simulink model "system_identification"  (R2024b)
settings: Solver=VariableStepAuto  StartTime=0.0  StopTime=1000  RelTol=1e-3
model workspace (MAT data in the model file):
  d = 0.5
  eps = 1
values from neighbouring files (symbols this model uses):
  s_L = slipRange(j)    [identify_system.m]
  s_R = slipRange(i)    [identify_system.m]
settings Model: Creator=radnor  LastModifiedBy=radnor

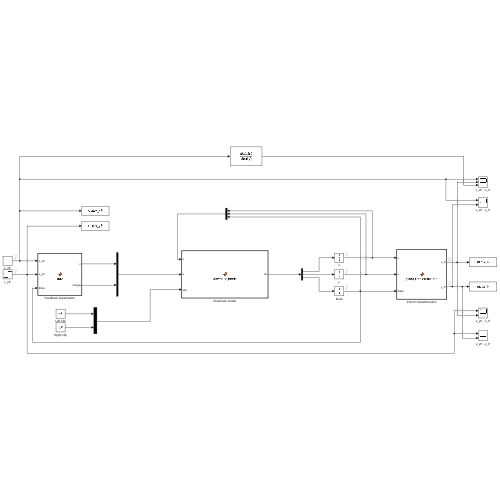
[thumbnail: Simulink's stored preview of the top-level diagram]
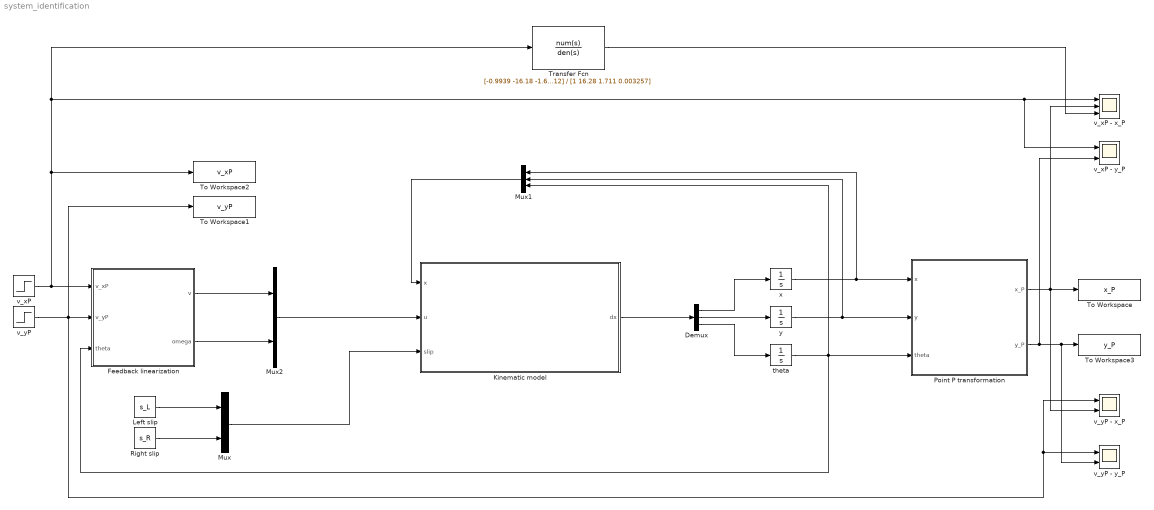
== system system_identification ==
  Demux : Demux  Outputs=3
  Feedback linearization : MATLAB Function  TreatAsAtomicUnit=on
  Kinematic model : MATLAB Function  TreatAsAtomicUnit=on
  Left slip : Constant  Value=s_L
  Mux : Mux  Inputs=2
  Mux1 : Mux  Inputs=3
  Mux2 : Mux  Inputs=2
  Point P transformation : MATLAB Function  TreatAsAtomicUnit=on
  Right slip : Constant  Value=s_R
  To Workspace : ToWorkspace  VariableName=x_P  SaveFormat=Timeseries  SampleTime=-1
  To Workspace1 : ToWorkspace  VariableName=v_yP  SaveFormat=Timeseries  SampleTime=-1
  To Workspace2 : ToWorkspace  VariableName=v_xP  SaveFormat=Timeseries  SampleTime=-1
  To Workspace3 : ToWorkspace  VariableName=y_P  SaveFormat=Timeseries  SampleTime=-1
  Transfer Fcn : TransferFcn  Numerator=[-0.9939 -16.18 -1.69 0.712]  Denominator=[1 16.28 1.711 0.003257]
  theta : Integrator
  v_xP : Step  Before=0.5  SampleTime=0
  v_xP - x_P : Scope  NumInputPorts=3
  v_xP - y_P : Scope  NumInputPorts=2
  v_yP : Step  Time=3  After=0.5  SampleTime=0
  v_yP - x_P : Scope  NumInputPorts=2
  v_yP - y_P : Scope  NumInputPorts=2
  x : Integrator
  y : Integrator
  wires:
  Mux/1 -> Kinematic model/3(slip)
  Demux/1 -> x/1
  Demux/2 -> y/1
  Demux/3 -> theta/1
  Kinematic model/1(dx) -> Demux/1
  x/1 -> Point P transformation/1(x), Mux1/1
  y/1 -> Point P transformation/2(y), Mux1/2
  theta/1 -> Mux1/3, Point P transformation/3(theta), Feedback linearization/3(theta)
  Mux1/1 -> Kinematic model/1(x)
  Feedback linearization/1(v) -> Mux2/1
  Feedback linearization/2(omega) -> Mux2/2
  Mux2/1 -> Kinematic model/2(u)
  v_yP/1 -> v_yP - y_P/1, v_yP - x_P/1, To Workspace1/1, Feedback linearization/2(v_yP)
  Point P transformation/1(x_P) -> v_yP - x_P/2, v_xP - x_P/2, To Workspace/1
  Point P transformation/2(y_P) -> v_yP - y_P/2, To Workspace3/1, v_xP - y_P/2
  Right slip/1 -> Mux/2
  Left slip/1 -> Mux/1
  Transfer Fcn/1 -> v_xP - x_P/3
  v_xP/1 -> Transfer Fcn/1, v_xP - y_P/1, v_xP - x_P/1, To Workspace2/1, Feedback linearization/1(v_xP)

== matlab function system_identification/Feedback linearization ==
  data: v_xP input; v output; v_yP input; theta input; omega output; eps parameter
function [v, omega] = ddv(v_xP, v_yP, theta, eps)
    v = v_xP*cos(theta)+v_yP*sin(theta);
    omega = -1/eps*sin(theta)*v_xP+1/eps*cos(theta)*v_yP;
end

== matlab function system_identification/Kinematic model ==
  data: x input size=3; u input; dx output size=3; slip input; d parameter
function dx = kinematic_model(x, u, slip, d)
    v = u(1);
    omega = u(2);

    theta = x(3);

    eta_L = 1-slip(1);
    eta_R = 1-slip(2);

    v_L = (v - d*omega) / eta_L;
    v_R = (v + d*omega) / eta_R;

    dx = zeros(3,1);
    dx(1) = 0.5*(eta_R*cos(theta)*v_R + eta_L*cos(theta)*v_L);
    dx(2) = 0.5*(eta_R*sin(theta)*v_R + eta_L*sin(theta)*v_L); 
    dx(3) = eta_R/(2*d)*v_R - eta_L/(2*d)*v_L;
end

== matlab function system_identification/Point P transformation ==
  data: x input; x_P output; y input; theta input; y_P output; eps parameter
function [x_P, y_P] = point_transformation(x, y, theta, eps)
    x_P = x + eps*cos(theta);
    y_P = y + eps*sin(theta);
end
